simulink model "q1_a2"  (R2022a)
settings: Solver=VariableStepAuto  StartTime=0.0  StopTime=40  RelTol=1e-3
settings Model: Creator=Asus  LastModifiedBy=ZahraIranpour
settings SolverCC: AlgebraicLoopSolver=TrustRegion
settings DataIOCC: ReturnWorkspaceOutputs=off
settings DebuggingCC: UnconnectedInputMsg=warning  UnconnectedOutputMsg=warning  UnconnectedLineMsg=warning  SFMachineParentedDataDiag=warning  ArithmeticOperatorsInVariantConditions=warning
settings SFSimCC: SimUseLocalCustomCode=off  CustomCodeUndefinedFunction=UseInterfaceOnly
settings RTWCC: RTWUseLocalCustomCode=off
settings CodeAppCC: StateflowObjectComments=on

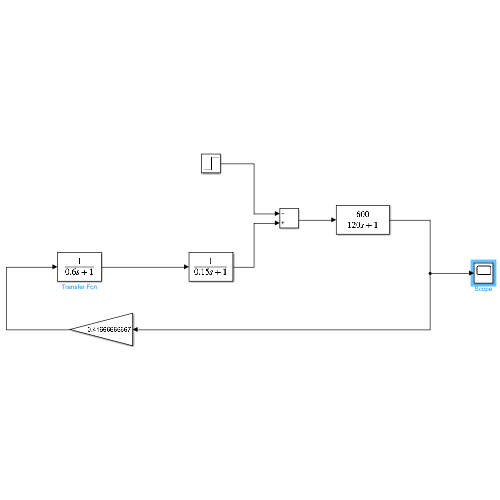
[thumbnail: Simulink's stored preview of the top-level diagram]
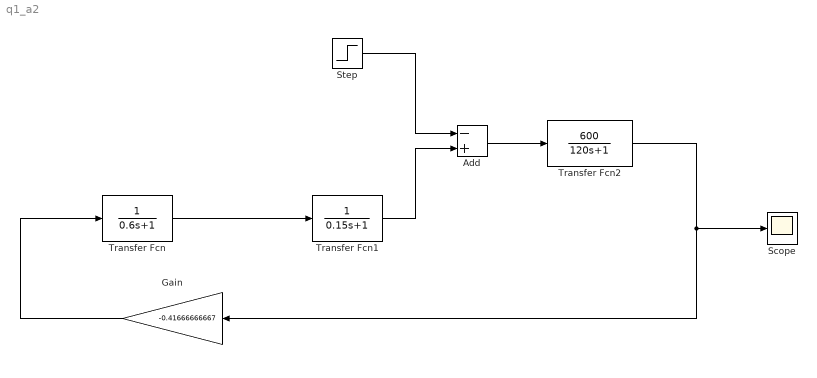
== system q1_a2 ==
  Add : Sum  Inputs=-+
  Gain : Gain  Gain=-0.41666666667
  Scope : Scope
  Step : Step  Time=0  After=0.2  SampleTime=0
  Transfer Fcn : TransferFcn  Denominator=[0.6 1]
  Transfer Fcn1 : TransferFcn  Denominator=[0.15 1]
  Transfer Fcn2 : TransferFcn  Numerator=[600]  Denominator=[120 1]
  wires:
  Transfer Fcn/1 -> Transfer Fcn1/1
  Transfer Fcn2/1 -> Scope/1, Gain/1
  Add/1 -> Transfer Fcn2/1
  Transfer Fcn1/1 -> Add/2
  Step/1 -> Add/1
  Gain/1 -> Transfer Fcn/1
